simulink model "Kapitsa_Pendulum"  (R2020a)
settings: Solver=VariableStepAuto  StartTime=0.0  StopTime=2  MaxStep=0.01  RelTol=1e-3
values from neighbouring files (symbols this model uses):
  A = 0.1    [intro.m]
  b = 0.1    [intro.m]
  l = 1    [intro.m]
  m = 1    [intro.m]
  startDegree = 10    [intro.m]
  w = 73    [intro.m]
libraries: simulink_extras x1, simulink x1
settings Model: EnablePacing=on  Creator=Gleb  LastModifiedBy=Gleb
settings DataIOCC: ReturnWorkspaceOutputs=off

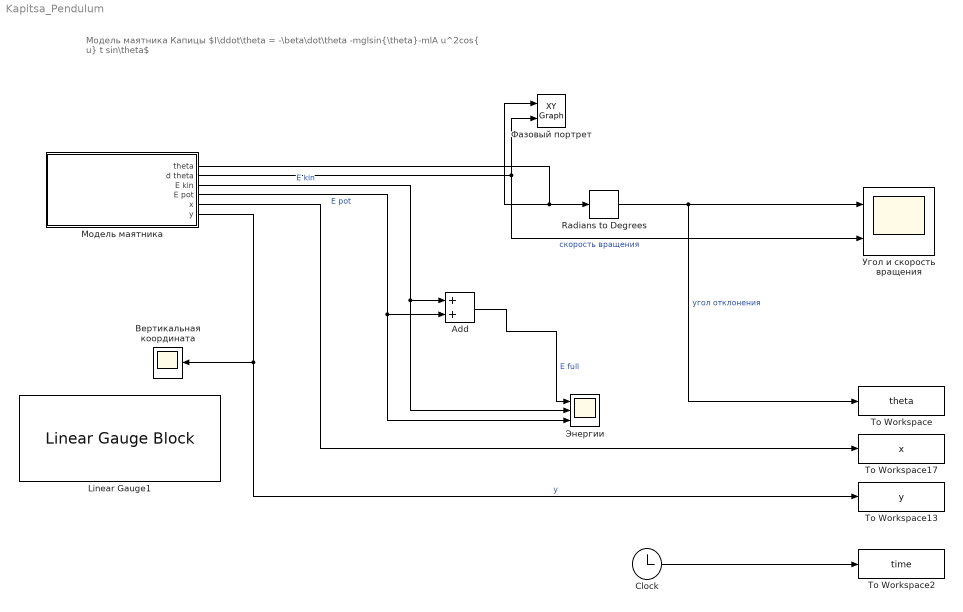
== system Kapitsa_Pendulum ==
  note: Модель маятника Капицы
      | $I\ddot\theta = -\beta\dot\theta -mglsin{\theta}-mlA\nu^2cos{\nu} t sin\theta$
  Add : Sum
  Clock : Clock
      settings: Decimation=2
  Linear Gauge1 : LinearGaugeBlock  ScaleMin=-2  ScaleMax=2  TickInterval=0.5
  Radians to Degrees : simulink_extras/Transformations/Radians to Degrees
  To Workspace : ToWorkspace  VariableName=theta  SampleTime=-1
      settings: Save2DSignal=2-D array (concatenate along first dimension)
  To Workspace13 : ToWorkspace  VariableName=y  SampleTime=-1
      settings: Save2DSignal=2-D array (concatenate along first dimension)
  To Workspace17 : ToWorkspace  VariableName=x  SampleTime=-1
      settings: Save2DSignal=2-D array (concatenate along first dimension)
  To Workspace2 : ToWorkspace  VariableName=time  SampleTime=-1
      settings: Save2DSignal=2-D array (concatenate along first dimension)
  Вертикальная координата : Scope
  Модель маятника : Subsystem  mask{m=m, l=l, g=9.8, startDegree=startDegree, b=b, A=A, w=w}
      mask prompts: m "Масса"; l "Длина нити"; g "Ускорение своб. падения"; startDegree "Стартовый угол, градусы"; b "Коэффициент сопротивления"; A "Амплитуда колебаний подвеса"; w "Частота собств. колебаний"
      mask init:
      | I = m* l^2
  Угол и скорость вращения : Scope  NumInputPorts=2
  Фазовый портрет : simulink/Sinks/XY Graph  xmin=-5  xmax=5  ymin=-5  ymax=5  st=-1
  Энергии : Scope  NumInputPorts=3
  wires:
  Radians to Degrees/1 -> Угол и скорость вращения/1, To Workspace/1  "угол отклонения"
  Модель маятника/1(theta) -> Фазовый портрет/1, Radians to Degrees/1
  Модель маятника/2(d theta) -> Фазовый портрет/2, Угол и скорость вращения/2  "скорость вращения"
  Модель маятника/4(E pot) -> Энергии/3, Add/2  "E pot"
  Модель маятника/3(E kin) -> Энергии/2, Add/1  "E kin"
  Add/1 -> Энергии/1  "E full"
  Модель маятника/6(y) -> To Workspace13/1, Вертикальная координата/1  "y"
  Модель маятника/5(x) -> To Workspace17/1
  Clock/1 -> To Workspace2/1

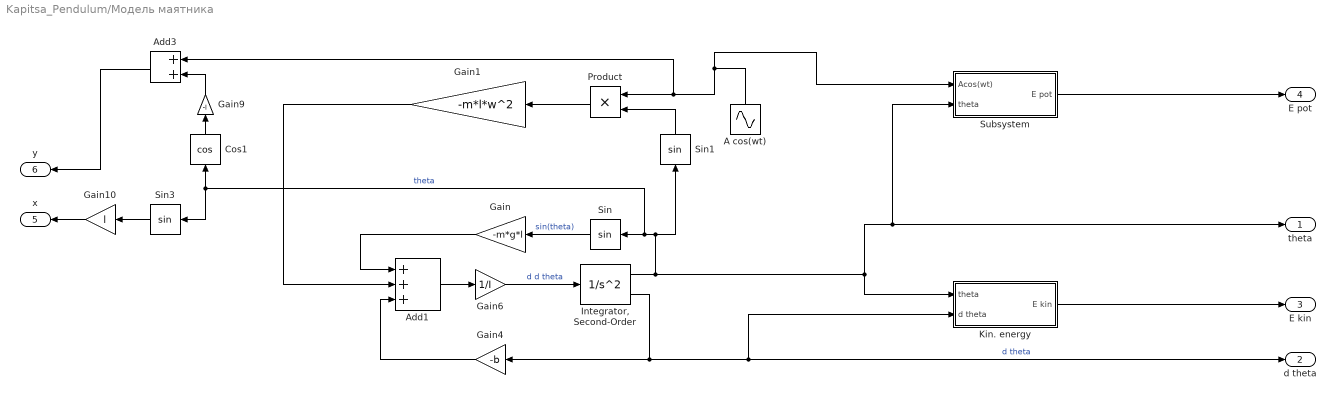
== system Kapitsa_Pendulum/Модель маятника ==
  A cos(wt) : Sin  Amplitude=A  Frequency=w  Phase=pi/2  SampleTime=0
  Add1 : Sum  Inputs=+++
  Add3 : Sum
  Cos1 : Trigonometry  Operator=cos
  Gain : Gain  Gain=-m*g*l
  Gain1 : Gain  Gain=-m*l*w^2
  Gain10 : Gain  Gain=l
  Gain4 : Gain  Gain=-b
  Gain6 : Gain  Gain=1/I
  Gain9 : Gain  Gain=-l
  "Integrator, Second-Order" : SecondOrderIntegrator  ICX=deg2rad(startDegree)
  Kin. energy : Subsystem
  Product : Product
  Sin : Trigonometry
  Sin1 : Trigonometry
  Sin3 : Trigonometry
  Subsystem : Subsystem
  theta : Outport
  d theta : Outport  Port=2
  E kin : Outport  Port=3
  E pot : Outport  Port=4
  x : Outport  Port=5
  y : Outport  Port=6
  wires:
  "Integrator, Second-Order"/1 -> Sin3/1, Cos1/1, Sin/1, Sin1/1, Subsystem/2(theta), theta/1, Kin. energy/1(theta)  "theta"
  "Integrator, Second-Order"/2 -> Kin. energy/2(d theta), d theta/1, Gain4/1  "d theta"
  Sin/1 -> Gain/1  "sin(theta)"
  Gain/1 -> Add1/1
  Gain6/1 -> "Integrator, Second-Order"/1  "d d theta"
  Add1/1 -> Gain6/1
  A cos(wt)/1 -> Add3/1, Product/1, Subsystem/1(Acos(wt))
  Product/1 -> Gain1/1
  Sin1/1 -> Product/2
  Gain4/1 -> Add1/3
  Gain1/1 -> Add1/2
  Kin. energy/1(E kin) -> E kin/1
  Cos1/1 -> Gain9/1
  Gain9/1 -> Add3/2
  Add3/1 -> y/1
  Sin3/1 -> Gain10/1
  Gain10/1 -> x/1
  Subsystem/1(E pot) -> E pot/1

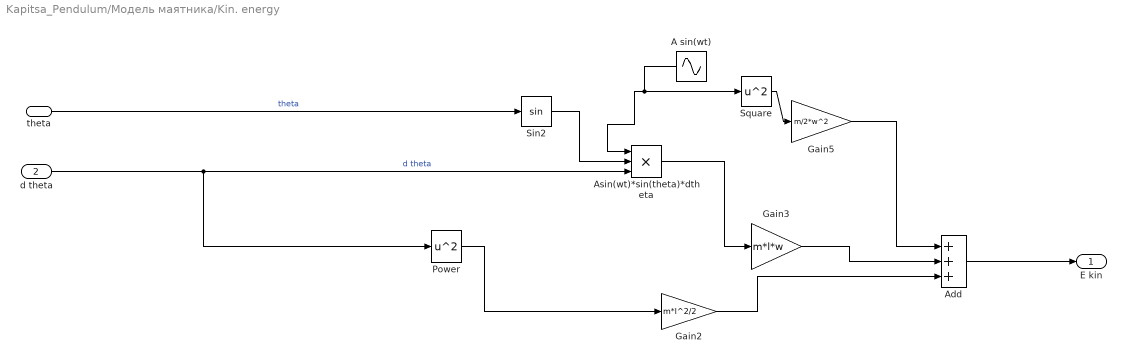
== system Kapitsa_Pendulum/Модель маятника/Kin. energy ==
  theta : Inport
  d theta : Inport  Port=2
  A sin(wt) : Sin  Amplitude=A  Frequency=w  SampleTime=0
  Add : Sum  Inputs=+++
  Asin(wt)*sin(theta)*dtheta : Product  Inputs=3
  Gain2 : Gain  Gain=m*l^2/2
  Gain3 : Gain  Gain=m*l*w
  Gain5 : Gain  Gain=m/2*w^2
  Power : Math  Operator=square  SaturateOnIntegerOverflow=on
  Sin2 : Trigonometry
  Square : Math  Operator=square  SaturateOnIntegerOverflow=on
  E kin : Outport
  wires:
  theta/1 -> Sin2/1  "theta"
  Add/1 -> E kin/1
  Gain3/1 -> Add/2
  Gain5/1 -> Add/1
  Sin2/1 -> Asin(wt)*sin(theta)*dtheta/2
  Square/1 -> Gain5/1
  Gain2/1 -> Add/3
  Power/1 -> Gain2/1
  Asin(wt)*sin(theta)*dtheta/1 -> Gain3/1
  d theta/1 -> Power/1, Asin(wt)*sin(theta)*dtheta/3  "d theta"
  A sin(wt)/1 -> Asin(wt)*sin(theta)*dtheta/1, Square/1

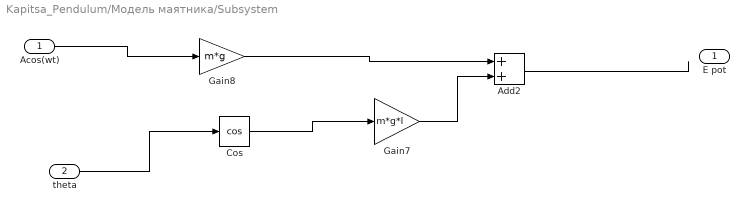
== system Kapitsa_Pendulum/Модель маятника/Subsystem ==
  Acos(wt) : Inport
  theta : Inport  Port=2
  Add2 : Sum
  Cos : Trigonometry  Operator=cos
  Gain7 : Gain  Gain=m*g*l
  Gain8 : Gain  Gain=m*g
  E pot : Outport
  wires:
  Gain8/1 -> Add2/1
  Add2/1 -> ?
  theta/1 -> Cos/1
  Gain7/1 -> Add2/2
  Cos/1 -> Gain7/1
  Acos(wt)/1 -> Gain8/1
